simulink model "chap1_4"  (R2016a)
settings: Solver=ode45  StartTime=0.0  StopTime=10.0  RelTol=1e-3
libraries: simulink x1
settings Model: Creator=admin  LastModifiedBy=admin

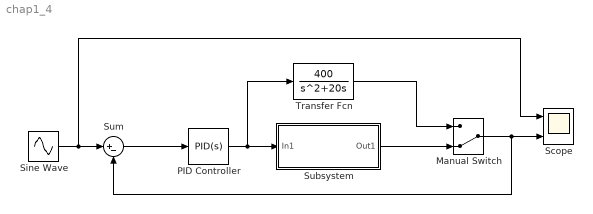
== system chap1_4 ==
  Manual Switch : ManualSwitch  CurrentSetting=0
  PID Controller : simulink/Continuous/PID Controller  Controller=PID  TimeDomain=Continuous-time  SampleTime=-1  IntegratorMethod=Forward Euler  FilterMethod=Forward Euler  Form=Parallel  UseFilter=on  ControllerParametersSource=internal  P=10  I=0  D=1  N=100  InitialConditionSource=internal  InitialConditionForIntegrator=0  InitialConditionForFilter=0  ExternalReset=none  LimitOutput=off  UpperSaturationLimit=inf  LowerSaturationLimit=-inf  LinearizeAsGain=on  AntiWindupMode=none  Kb=1  TrackingMode=off  Kt=1  PParamMin=[]  PParamMax=[]  IParamMin=[]  IParamMax=[]  DParamMin=[]  DParamMax=[]  NParamMin=[]  NParamMax=[]  KbParamMin=[]  KbParamMax=[]  KtParamMin=[]  KtParamMax=[]  POutMin=[]  POutMax=[]  IOutMin=[]  IOutMax=[]  DOutMin=[]  DOutMax=[]  NOutMin=[]  NOutMax=[]  KbOutMin=[]  KbOutMax=[]  KtOutMin=[]  KtOutMax=[]  IntegratorOutMin=[]  IntegratorOutMax=[]  FilterOutMin=[]  FilterOutMax=[]  SumOutMin=[]  SumOutMax=[]  SumI1OutMin=[]  SumI1OutMax=[]  SumI2OutMin=[]  SumI2OutMax=[]  SumI3OutMin=[]  SumI3OutMax=[]  SumDOutMin=[]  SumDOutMax=[]  SaturationOutMin=[]  SaturationOutMax=[]  IntegratorContinuousStateAttributes=''  IntegratorStateMustResolveToSignalObject=off  IntegratorRTWStateStorageClass=Auto  FilterContinuousStateAttributes=''  FilterStateMustResolveToSignalObject=off  FilterRTWStateStorageClass=Auto  DifferentiatorICPrevScaledInput=0  DifferentiatorOutMin=[]  DifferentiatorOutMax=[]
  Scope : Scope  NumInputPorts=2
  Sine Wave : Sin  Amplitude=0.5  Frequency=2*pi  SampleTime=0
  Subsystem : Subsystem
  Sum : Sum  Inputs=|+-
  Transfer Fcn : TransferFcn  Numerator=[400]  Denominator=[1 20 0]
  wires:
  Sine Wave/1 -> Scope/1, Sum/1
  Subsystem/1(Out1) -> Manual Switch/2
  Sum/1 -> PID Controller/1
  PID Controller/1 -> Transfer Fcn/1, Subsystem/1(In1)
  Transfer Fcn/1 -> Manual Switch/1
  Manual Switch/1 -> Sum/2, Scope/2

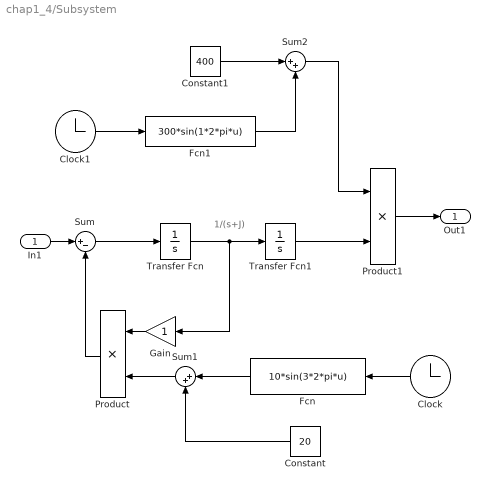
== system chap1_4/Subsystem ==
  note: 1/(s+J)
  In1 : Inport
  Clock : Clock
  Clock1 : Clock
  Constant : Constant  Value=20
  Constant1 : Constant  Value=400
  Fcn : Fcn  Expr=10*sin(3*2*pi*u)
  Fcn1 : Fcn  Expr=300*sin(1*2*pi*u)
  Gain : Gain
  Product : Product
  Product1 : Product
  Sum : Sum  Inputs=|+-
  Sum1 : Sum  Inputs=|++
  Sum2 : Sum  Inputs=|++
  Transfer Fcn : TransferFcn  Denominator=[1 0]
  Transfer Fcn1 : TransferFcn  Denominator=[1 0]
  Out1 : Outport
  wires:
  In1/1 -> Sum/1
  Sum/1 -> Transfer Fcn/1
  Gain/1 -> Product/1
  Sum1/1 -> Product/2
  Fcn/1 -> Sum1/1
  Clock/1 -> Fcn/1
  Constant/1 -> Sum1/2
  Transfer Fcn/1 -> Transfer Fcn1/1, Gain/1
  Product/1 -> Sum/2
  Clock1/1 -> Fcn1/1
  Constant1/1 -> Sum2/1
  Fcn1/1 -> Sum2/2
  Transfer Fcn1/1 -> Product1/2
  Sum2/1 -> Product1/1
  Product1/1 -> Out1/1
